simulink model "sampleModel1498"  (R2023a)
settings: Solver=VariableStepAuto  StartTime=0.0  StopTime=10.0  RelTol=1e-3
libraries: hdlsllib x7
settings Model: Creator=user1  LastModifiedBy=user1

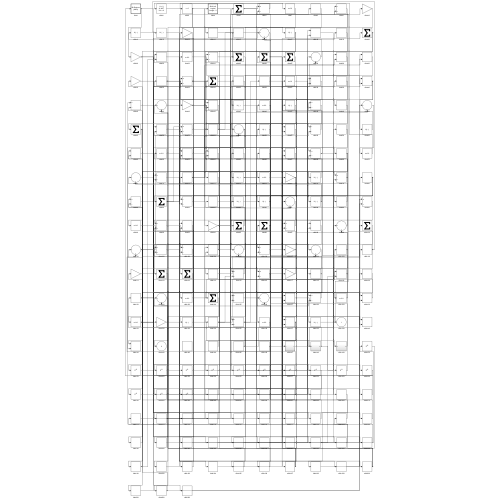
[thumbnail: Simulink's stored preview of the top-level diagram]
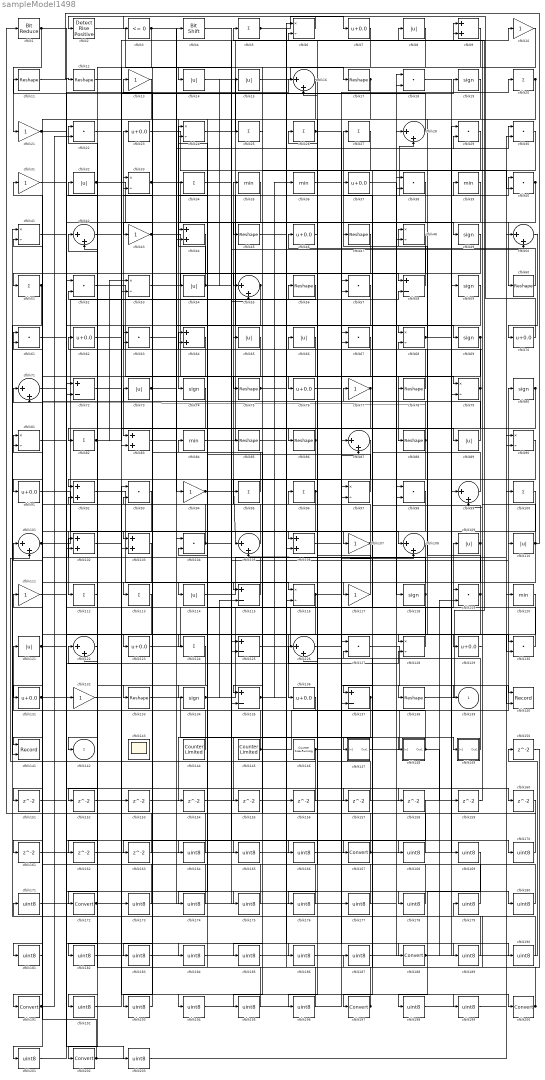
== system sampleModel1498 ==
  cfblk1 : hdlsllib/Logic and Bit Operations/Bit Reduce  mode=AND
  cfblk{10,13,21,31,43,77,94,107,111,117,132} (11 alike) : Gain
  cfblk{5,20,25..27,34,51,82,95..96,100,112..113,124} (14 alike) : Sum  Inputs=+
  cfblk{16,28,42,50,55,71,87,99,101,105,108,122,126} (13 alike) : Sum  Inputs=|++
  cfblk{9,44,64,83,92,102..103,106} (8 alike) : Sum
  cfblk{18,22,29..30,38,40,52,57,61,63,67,93,98,104,119,127,130} (17 alike) : DotProduct  OutDataTypeStr=Inherit: Inherit via internal rule
  cfblk{8,14..15,32,54,65..66,73,89,109..110,114,121} (13 alike) : Abs  SaturateOnIntegerOverflow=off
  cfblk{11..12,17,45,47,56,60,75,78,85..86,88,133,138} (14 alike) : Reshape
  cfblk{58,72,115,125,135,137} (6 alike) : Sum  Inputs=+-
  cfblk{6,24,33,41,48,53,68,79,81,90,97,116,128} (13 alike) : Product  Inputs=*/  RndMeth=Zero  SaturateOnIntegerOverflow=on
  cfblk{19,49,59,69,74,80,118,134} (8 alike) : Signum
  cfblk{35..36,39,84,120} (5 alike) : MinMax
  cfblk{7,23,37,46,62,70,76,91,123,129,131,136} (12 alike) : Bias  Bias=0.0  SaturateOnIntegerOverflow=off
  cfblk140 : Record  FileSettingsInternal="{\"entries\":[{\"content\":{\"excelSettings\":{\"content\":{},\"type\":\"Streamout.ExcelSettings\"}},\"type\":\"Streamout.FileSettingStorage\",\"uuid\":\"\"}],\"packageUris\":[\"http:\\/\\/schema.mathworks.com\\/mf0\\/streamout_blocks\\/R2020a\"],\"version\":\"1.0\"}"  Layout=[1 1]  SignalsInternal="{\"entries\":[{\"content\":{\"signals\":[{\"content\":{\"blockPath\":[],\"dimensions\":[1],\"domain\":\"\",\"lineColor\":\"#a2142f\",\"plots\":[1],\"port\":1,\"signalID\":1241,\"signalName\":\"XY Graph:1\"},\"type\":\"RecordBlkView.Signal\",\"uuid\":\"\"},{\"content\":{\"blockPath\":[],\"dimensions\":[1],\"domain\":\"\",\"lineColor\":\"#139fff\",\"plots\":[1],\"port\":2,\"signalID\":1244,\"signalName\":\"XY Graph:2\"},\"type\":\"RecordBlkView.Signal\",\"uuid\":\"\"}]},\"type\":\"RecordBlkView.InputSignals\",\"uuid\":\"\"}],\"packageUris\":[\"http:\\/\\/schema.mathworks.com\\/mf0\\/streamout_blocks\\/R2020a\"],\"version\":\"1.0\"}"  VisualizationBindings="{\"xyplotplugin\":{\"info\":[{\"series\":[{\"bindingParametersList\":[{\"parameter\":\"X-Axis\",\"signalID\":1241,\"signalName\":\"XY Graph:1\"},{\"parameter\":\"Y-Axis\",\"signalID\":1244,\"signalName\":\"XY Graph:2\"}],\"seriesID\":14841}],\"subplotID\":1}]}}"  CompatibilityTag=XY  st=-1
  cfblk141 : Record  FileSettingsInternal="{\"entries\":[{\"content\":{\"excelSettings\":{\"content\":{},\"type\":\"Streamout.ExcelSettings\"}},\"type\":\"Streamout.FileSettingStorage\",\"uuid\":\"\"}],\"packageUris\":[\"http:\\/\\/schema.mathworks.com\\/mf0\\/streamout_blocks\\/R2020a\"],\"version\":\"1.0\"}"  Layout=[1 1]  SignalsInternal="{\"entries\":[{\"content\":{\"signals\":[{\"content\":{\"blockPath\":[],\"dimensions\":[1],\"domain\":\"\",\"lineColor\":\"#a2142f\",\"plots\":[1],\"port\":1,\"signalID\":1249,\"signalName\":\"XY Graph:1\"},\"type\":\"RecordBlkView.Signal\",\"uuid\":\"\"},{\"content\":{\"blockPath\":[],\"dimensions\":[1],\"domain\":\"\",\"lineColor\":\"#139fff\",\"plots\":[1],\"port\":2,\"signalID\":1252,\"signalName\":\"XY Graph:2\"},\"type\":\"RecordBlkView.Signal\",\"uuid\":\"\"}]},\"type\":\"RecordBlkView.InputSignals\",\"uuid\":\"\"}],\"packageUris\":[\"http:\\/\\/schema.mathworks.com\\/mf0\\/streamout_blocks\\/R2020a\"],\"version\":\"1.0\"}"  VisualizationBindings="{\"xyplotplugin\":{\"info\":[{\"series\":[{\"bindingParametersList\":[{\"parameter\":\"X-Axis\",\"signalID\":1249,\"signalName\":\"XY Graph:1\"},{\"parameter\":\"Y-Axis\",\"signalID\":1252,\"signalName\":\"XY Graph:2\"}],\"seriesID\":4770}],\"subplotID\":1}]}}"  CompatibilityTag=XY  st=-1
  cfblk143 : Scope
      settings: Floating=on
  cfblk144 : hdlsllib/Sources/Counter Limited  uplimit=7  tsamp=-1
  cfblk145 : hdlsllib/Sources/Counter Limited  uplimit=7  tsamp=-1
  cfblk146 : hdlsllib/Sources/Counter Free-Running  NumBits=16  tsamp=-1
  cfblk147 : Subsystem
      settings: LibrarySourceBlock=|
      | hdlsllib/Ports &
      | Subsystems/Subsystem
  cfblk148 : Subsystem
      settings: LibrarySourceBlock=|
      | hdlsllib/Ports &
      | Subsystems/Subsystem
  cfblk149 : Subsystem
      settings: LibrarySourceBlock=|
      | hdlsllib/Ports &
      | Subsystems/Subsystem
  cfblk{150..163} (14 alike) : Delay  SampleTime=1
  cfblk{164..166,168..171,173..187,189..190,192..196,198..199,201,203} (33 alike) : DataTypeConversion  OutDataTypeStr=uint8  SaturateOnIntegerOverflow=off  RndMeth=Floor
  cfblk{167,172,188,191,197,200,202} (7 alike) : DataTypeConversion  SaturateOnIntegerOverflow=off  RndMeth=Floor
  cfblk2 : hdlsllib/Logic and Bit Operations/Detect Rise Positive  vinit=0  OutDataTypeStr=boolean
  cfblk3 : hdlsllib/Logic and Bit Operations/Compare To Zero  relop=<=  OutDataTypeStr=boolean
  cfblk4 : hdlsllib/Logic and Bit Operations/Bit Shift  mode=Shift Left Logical  N=0
  cfblk139 : Outport  VectorParamsAs1DForOutWhenUnconnected=off
  cfblk142 : Outport  Port=2  VectorParamsAs1DForOutWhenUnconnected=off
  wires:
  cfblk17/1 -> cfblk74/1, cfblk83/2
  cfblk99/1 -> cfblk61/1
  cfblk92/1 -> cfblk116/1
  cfblk57/1 -> cfblk83/1
  cfblk116/1 -> cfblk138/1, cfblk195/1
  cfblk134/1 -> cfblk96/1, cfblk115/2, cfblk110/1
  cfblk32/1 -> cfblk49/1, cfblk57/2
  cfblk83/1 -> cfblk4/1
  cfblk137/1 -> cfblk154/1, cfblk155/1
  cfblk125/1 -> cfblk109/1
  cfblk138/1 -> cfblk5/1
  cfblk55/1 -> cfblk113/1, cfblk72/2
  cfblk69/1 -> cfblk88/1, cfblk115/1
  cfblk104/1 -> cfblk22/1, cfblk29/2
  cfblk70/1 -> cfblk2/1
  cfblk147/1(Out1) -> cfblk80/1
  cfblk77/1 -> cfblk106/1, cfblk124/1
  cfblk43/1 -> cfblk76/1, cfblk125/2
  cfblk149/1(Out1) -> cfblk66/1
  cfblk53/1 -> cfblk58/1
  cfblk14/1 -> cfblk69/1
  cfblk52/1 -> cfblk79/1
  cfblk58/1 -> cfblk27/1
  cfblk120/1 -> cfblk136/1
  cfblk68/1 -> cfblk48/1, cfblk140/2
  cfblk105/1 -> cfblk35/1
  cfblk89/1 -> cfblk37/1
  cfblk33/1 -> cfblk48/2, cfblk68/1
  cfblk24/1 -> cfblk9/1
  cfblk101/1 -> cfblk58/2, cfblk130/1
  cfblk1/1 -> cfblk21/1, cfblk44/2
  cfblk5/1 -> cfblk7/1, cfblk40/2
  cfblk40/1 -> cfblk60/1, cfblk137/2
  cfblk29/1 -> cfblk147/1(In1)
  cfblk60/1 -> cfblk46/1
  cfblk26/1 -> cfblk140/1, cfblk189/1
  cfblk97/1 -> cfblk64/1
  cfblk78/1 -> cfblk23/1
  cfblk39/1 -> cfblk117/1
  cfblk136/1 -> cfblk121/1
  cfblk122/1 -> cfblk172/1
  cfblk84/1 -> cfblk28/2
  cfblk9/1 -> cfblk43/1
  cfblk128/1 -> cfblk47/1
  cfblk35/1 -> cfblk114/1
  cfblk131/1 -> cfblk119/1, cfblk128/2, cfblk39/1
  cfblk96/1 -> cfblk112/1, cfblk6/2, cfblk133/1
  cfblk80/1 -> cfblk82/1, cfblk106/2, cfblk166/1
  cfblk117/1 -> cfblk26/1
  cfblk109/1 -> cfblk77/1, cfblk137/1
  cfblk144/1 -> cfblk81/1
  cfblk13/1 -> cfblk51/1
  cfblk25/1 -> cfblk135/1
  cfblk4/1 -> cfblk97/2
  cfblk8/1 -> cfblk14/1
  cfblk91/1 -> cfblk107/1
  cfblk90/1 -> cfblk197/1
  cfblk45/1 -> cfblk129/1
  cfblk54/1 -> cfblk24/1, cfblk15/1, cfblk50/2
  cfblk115/1 -> cfblk102/1
  cfblk133/1 -> cfblk148/1(In1)
  cfblk82/1 -> cfblk19/1, cfblk8/1, cfblk53/1
  cfblk146/1 -> cfblk101/2, cfblk108/2
  cfblk108/1 -> cfblk134/1
  cfblk21/1 -> cfblk130/2, cfblk168/1
  cfblk100/1 -> cfblk202/1
  cfblk50/1 -> cfblk70/1
  cfblk118/1 -> cfblk61/2, cfblk181/1
  cfblk15/1 -> cfblk17/1
  cfblk2/1 -> cfblk135/2
  cfblk135/1 -> cfblk36/1, cfblk190/1
  cfblk56/1 -> cfblk52/2
  cfblk36/1 -> cfblk149/1(In1)
  cfblk49/1 -> cfblk55/1
  cfblk44/1 -> cfblk91/1
  cfblk47/1 -> cfblk75/1
  cfblk103/1 -> cfblk141/1
  cfblk94/1 -> cfblk105/1, cfblk10/1
  cfblk20/1 -> cfblk128/1, cfblk102/2
  cfblk76/1 -> cfblk108/1
  cfblk27/1 -> cfblk45/1
  cfblk148/1(Out1) -> cfblk33/2, cfblk159/1
  cfblk121/1 -> cfblk72/1, cfblk33/1
  cfblk73/1 -> cfblk30/1, cfblk40/1
  cfblk123/1 -> cfblk25/1
  cfblk37/1 -> cfblk118/1
  cfblk3/1 -> cfblk94/1, cfblk142/1, cfblk53/2
  cfblk63/1 -> cfblk56/1
  cfblk129/1 -> cfblk99/2
  cfblk106/1 -> cfblk20/1
  cfblk114/1 -> cfblk30/2
  cfblk28/1 -> cfblk11/1
  cfblk41/1 -> cfblk188/1
  cfblk88/1 -> cfblk95/1, cfblk62/1, cfblk71/2
  cfblk51/1 -> cfblk131/1, cfblk141/2
  cfblk48/1 -> cfblk103/1
  cfblk145/1 -> cfblk59/1, cfblk104/2
  cfblk59/1 -> cfblk63/1
  cfblk81/1 -> cfblk16/1
  cfblk127/1 -> cfblk139/1
  cfblk12/1 -> cfblk89/1
  cfblk75/1 -> cfblk78/1, cfblk157/1
  cfblk85/1 -> cfblk167/1
  cfblk66/1 -> cfblk116/2
  cfblk79/1 -> cfblk32/1, cfblk92/1
  cfblk107/1 -> cfblk105/2, cfblk71/1
  cfblk6/1 -> cfblk3/1
  cfblk93/1 -> cfblk191/1
  cfblk110/1 -> cfblk12/1, cfblk123/1, cfblk68/2
  cfblk132/1 -> cfblk200/1
  cfblk95/1 -> cfblk73/1
  cfblk130/1 -> cfblk34/1
  cfblk16/1 -> cfblk44/1
  cfblk65/1 -> cfblk103/2
  cfblk19/1 -> cfblk86/1
  cfblk86/1 -> cfblk64/2, cfblk174/1
  cfblk119/1 -> cfblk65/1, cfblk152/1
  cfblk67/1 -> cfblk151/1
  cfblk72/1 -> cfblk153/1
  cfblk153/1 -> cfblk55/2
  cfblk154/1 -> cfblk28/1
  cfblk155/1 -> cfblk79/2
  cfblk23/1 -> cfblk156/1
  cfblk156/1 -> cfblk24/2
  cfblk157/1 -> cfblk16/2
  cfblk71/1 -> cfblk158/1
  cfblk159/1 -> cfblk9/2
  cfblk102/1 -> cfblk160/1
  cfblk160/1 -> cfblk1/1
  cfblk64/1 -> cfblk161/1
  cfblk161/1 -> cfblk97/1
  cfblk124/1 -> cfblk162/1
  cfblk162/1 -> cfblk29/1
  cfblk74/1 -> cfblk163/1
  cfblk163/1 -> cfblk52/1
  cfblk38/1 -> cfblk164/1
  cfblk164/1 -> cfblk101/1
  cfblk10/1 -> cfblk165/1
  cfblk165/1 -> cfblk38/1
  cfblk166/1 -> cfblk38/2
  cfblk167/1 -> cfblk63/2, cfblk127/1
  cfblk168/1 -> cfblk85/1
  cfblk18/1 -> cfblk169/1
  cfblk34/1 -> cfblk170/1
  cfblk170/1 -> cfblk18/1
  cfblk171/1 -> cfblk18/2
  cfblk172/1 -> cfblk125/1, cfblk54/1
  cfblk62/1 -> cfblk173/1
  cfblk173/1 -> cfblk122/1
  cfblk174/1 -> cfblk122/2
  cfblk31/1 -> cfblk175/1
  cfblk175/1 -> cfblk13/1
  cfblk30/1 -> cfblk176/1
  cfblk176/1 -> cfblk31/1
  cfblk126/1 -> cfblk177/1
  cfblk177/1 -> cfblk104/1
  cfblk151/1 -> cfblk178/1
  cfblk178/1 -> cfblk126/1
  cfblk179/1 -> cfblk126/2
  cfblk111/1 -> cfblk180/1
  cfblk180/1 -> cfblk57/1
  cfblk181/1 -> cfblk111/1
  cfblk87/1 -> cfblk182/1
  cfblk182/1 -> cfblk150/1
  cfblk7/1 -> cfblk183/1
  cfblk183/1 -> cfblk87/1
  cfblk61/1 -> cfblk184/1
  cfblk184/1 -> cfblk87/2
  cfblk98/1 -> cfblk185/1
  cfblk185/1 -> cfblk99/1
  cfblk22/1 -> cfblk186/1
  cfblk186/1 -> cfblk98/1
  cfblk150/1 -> cfblk187/1
  cfblk187/1 -> cfblk98/2
  cfblk188/1 -> cfblk120/1, cfblk119/2
  cfblk189/1 -> cfblk41/1
  cfblk190/1 -> cfblk41/2
  cfblk191/1 -> cfblk171/1, cfblk22/2
  cfblk112/1 -> cfblk192/1
  cfblk192/1 -> cfblk93/1
  cfblk158/1 -> cfblk193/1
  cfblk193/1 -> cfblk93/2
  cfblk42/1 -> cfblk194/1
  cfblk194/1 -> cfblk67/2
  cfblk195/1 -> cfblk42/1
  cfblk46/1 -> cfblk196/1
  cfblk196/1 -> cfblk42/2
  cfblk197/1 -> cfblk92/2, cfblk84/1, cfblk67/1
  cfblk169/1 -> cfblk198/1
  cfblk198/1 -> cfblk90/1
  cfblk152/1 -> cfblk199/1
  cfblk199/1 -> cfblk90/2
  cfblk200/1 -> cfblk179/1, cfblk127/2, cfblk6/1
  cfblk113/1 -> cfblk201/1
  cfblk201/1 -> cfblk132/1
  cfblk202/1 -> cfblk81/2, cfblk50/1
  cfblk11/1 -> cfblk203/1
  cfblk203/1 -> cfblk100/1

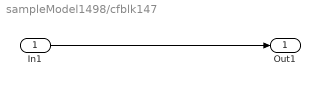
== system sampleModel1498/cfblk147 ==
  In1 : Inport
  Out1 : Outport
  wires:
  In1/1 -> Out1/1

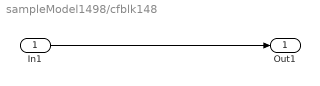
== system sampleModel1498/cfblk148 ==
  In1 : Inport
  Out1 : Outport
  wires:
  In1/1 -> Out1/1

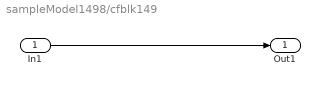
== system sampleModel1498/cfblk149 ==
  In1 : Inport
  Out1 : Outport
  wires:
  In1/1 -> Out1/1
